simulink library "SlewAndControlConstrained_Controller_lib"  (R2018b)
settings: Solver=VariableStepAuto  StartTime=0.0  StopTime=10.0  RelTol=1e-3
undefined symbols (not defined in the file or in its folder): fswParams
libraries: two_norm x2, aerolibutil x2, dspmtrx3 x1
settings Model: Creator=colem  LastModifiedBy=colem

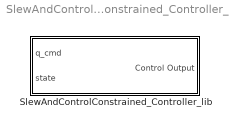
== system SlewAndControlConstrained_Controller_lib ==
  SlewAndControlConstrained_Controller_lib : Subsystem

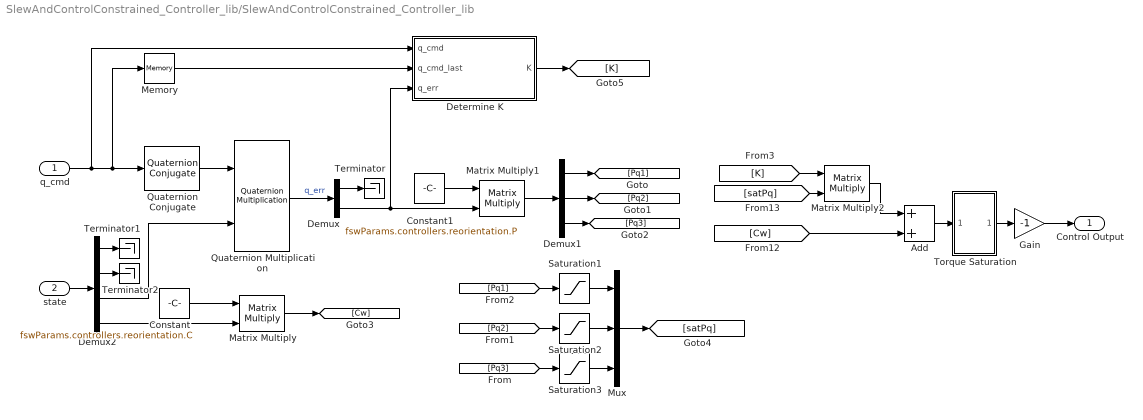
== system SlewAndControlConstrained_Controller_lib/SlewAndControlConstrained_Controller_lib ==
  q_cmd : Inport
  state : Inport  Port=2
  Add : Sum
  Constant : Constant  Value=fswParams.controllers.reorientation.C
  Constant1 : Constant  Value=fswParams.controllers.reorientation.P
  Demux : Demux  Outputs=[1 3]
  Demux1 : Demux  Outputs=3
  Demux2 : Demux  Outputs=[3 3 4 3]
  Determine K : Subsystem
  Gain : Gain  Gain=-1
  Matrix Multiply : Product  Multiplication=Matrix(*)
  Matrix Multiply1 : Product  Multiplication=Matrix(*)
  Matrix Multiply2 : Product  Multiplication=Matrix(*)
  Memory : Memory  InitialCondition=[.5;.5;.5;.5]  InheritSampleTime=on
  Mux : Mux  Inputs=3
  Quaternion Conjugate : aerolibutil/Quaternion Conjugate
      settings: SourceProductName=Aerospace Blockset  SourceProductBaseCode=AE
  Quaternion Multiplication : aerolibutil/Quaternion Multiplication
  Saturation1 : Saturate  UpperLimit=fswParams.controllers.reorientation.saturation  LowerLimit=-fswParams.controllers.reorientation.saturation
  Saturation2 : Saturate  UpperLimit=fswParams.controllers.reorientation.saturation  LowerLimit=-fswParams.controllers.reorientation.saturation
  Saturation3 : Saturate  UpperLimit=fswParams.controllers.reorientation.saturation  LowerLimit=-fswParams.controllers.reorientation.saturation
  Terminator : Terminator
  Terminator1 : Terminator
  Terminator2 : Terminator
  Torque Saturation : Subsystem
  Control Output : Outport
  wires:
  Quaternion Conjugate/1 -> Quaternion Multiplication/1
  Constant1/1 -> Matrix Multiply1/1
  Demux1/3 -> [Pq3]
  Matrix Multiply1/1 -> Demux1/1
  Matrix Multiply/1 -> [Cw]
  Demux1/1 -> [Pq1]
  q_cmd/1 -> Determine K/1(q_cmd), Memory/1, Quaternion Conjugate/1
  Constant/1 -> Matrix Multiply/1
  Demux1/2 -> [Pq2]
  Demux/1 -> Terminator/1
  Quaternion Multiplication/1 -> Demux/1  "q_err"
  Demux/2 -> Matrix Multiply1/2, Determine K/3(q_err)
  [Pq1] -> Saturation1/1
  [Pq2] -> Saturation2/1
  [Pq3] -> Saturation3/1
  [satPq] -> Matrix Multiply2/2
  [Cw] -> Add/2
  Torque Saturation/1(Out1) -> Gain/1
  Gain/1 -> Control Output/1
  Add/1 -> Torque Saturation/1(In1)
  Matrix Multiply2/1 -> Add/1
  state/1 -> Demux2/1
  Demux2/1 -> Terminator1/1
  Demux2/2 -> Terminator2/1
  Demux2/3 -> Quaternion Multiplication/2
  Demux2/4 -> Matrix Multiply/2
  Saturation1/1 -> Mux/1
  Saturation2/1 -> Mux/2
  Saturation3/1 -> Mux/3
  Mux/1 -> [satPq]
  Determine K/1(K) -> [K]
  Memory/1 -> Determine K/2(q_cmd_last)
  [K] -> Matrix Multiply2/1

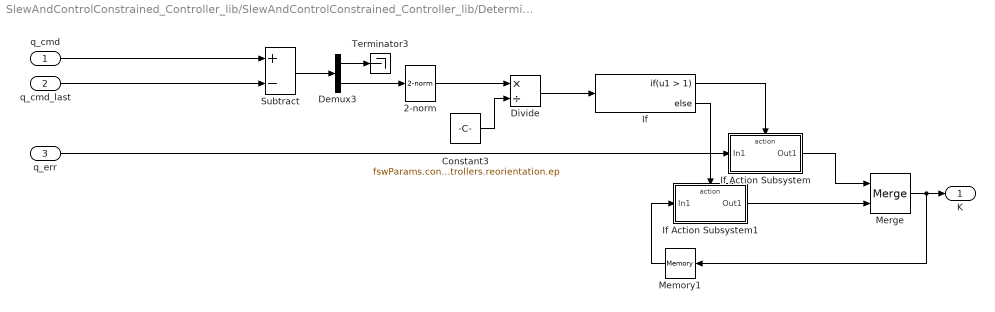
== system SlewAndControlConstrained_Controller_lib/SlewAndControlConstrained_Controller_lib/Determine K ==
  q_cmd : Inport
  q_cmd_last : Inport  Port=2
  q_err : Inport  Port=3
  2-norm : two_norm/2-norm  SystemSampleTime=-1
  Constant3 : Constant  Value=fswParams.controllers.reorientation.ep
  Demux3 : Demux  Outputs=[1 3]
  Divide : Product  Inputs=*/
  If : If  IfExpression=u1 > 1
  If Action Subsystem : Subsystem  TreatAsAtomicUnit=on
  If Action Subsystem1 : Subsystem  TreatAsAtomicUnit=on
  Memory1 : Memory  InitialCondition=fswParams.controllers.reorientation.K_init  InheritSampleTime=on
  Merge : Merge
  Subtract : Sum  Inputs=+-
  Terminator3 : Terminator
  K : Outport
  wires:
  Demux3/2 -> 2-norm/1
  If Action Subsystem/1(Out1) -> Merge/1
  If/1 -> If Action Subsystem/Action
  Divide/1 -> If/1
  q_err/1 -> If Action Subsystem/1(In1)
  2-norm/1 -> Divide/1
  Memory1/1 -> If Action Subsystem1/1(In1)
  Constant3/1 -> Divide/2
  If/2 -> If Action Subsystem1/Action
  If Action Subsystem1/1(Out1) -> Merge/2
  Demux3/1 -> Terminator3/1
  Subtract/1 -> Demux3/1
  Merge/1 -> Memory1/1, K/1
  q_cmd/1 -> Subtract/1
  q_cmd_last/1 -> Subtract/2

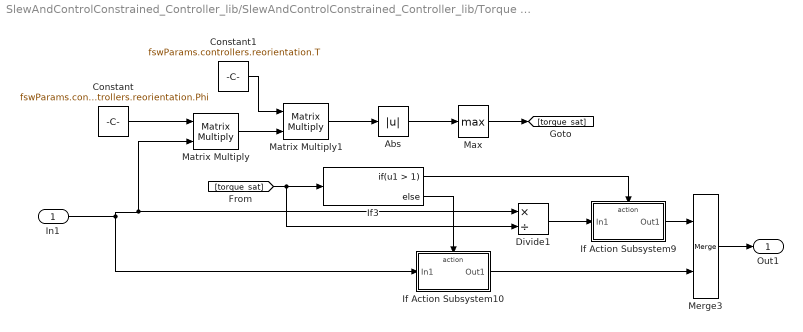
== system SlewAndControlConstrained_Controller_lib/SlewAndControlConstrained_Controller_lib/Torque Saturation ==
  In1 : Inport
  Abs : Abs
  Constant : Constant  Value=fswParams.controllers.reorientation.Phi
  Constant1 : Constant  Value=fswParams.controllers.reorientation.T
  Divide1 : Product  Inputs=*/
  If Action Subsystem10 : Subsystem  TreatAsAtomicUnit=on
  If Action Subsystem9 : Subsystem  TreatAsAtomicUnit=on
  If3 : If  IfExpression=u1 > 1
  Matrix Multiply : Product  Multiplication=Matrix(*)
  Matrix Multiply1 : Product  Multiplication=Matrix(*)
  Max : MinMax  Function=max
  Merge3 : Merge
  Out1 : Outport
  wires:
  If Action Subsystem9/1(Out1) -> Merge3/1
  If3/1 -> If Action Subsystem9/Action
  If3/2 -> If Action Subsystem10/Action
  If Action Subsystem10/1(Out1) -> Merge3/2
  Merge3/1 -> Out1/1
  Divide1/1 -> If Action Subsystem9/1(In1)
  Constant/1 -> Matrix Multiply/1
  In1/1 -> Matrix Multiply/2, Divide1/1, If Action Subsystem10/1(In1)
  Matrix Multiply/1 -> Matrix Multiply1/2
  Constant1/1 -> Matrix Multiply1/1
  Matrix Multiply1/1 -> Abs/1
  Abs/1 -> Max/1
  [torque_sat] -> Divide1/2, If3/1
  Max/1 -> [torque_sat]

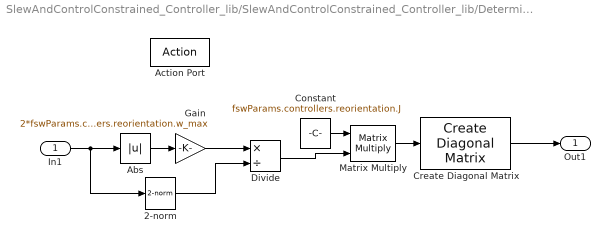
== system SlewAndControlConstrained_Controller_lib/SlewAndControlConstrained_Controller_lib/Determine K/If Action Subsystem ==
  In1 : Inport
  Action Port : ActionPort  ActionType=then
  2-norm : two_norm/2-norm  SystemSampleTime=-1
  Abs : Abs
  Constant : Constant  Value=fswParams.controllers.reorientation.J
  Create Diagonal Matrix : dspmtrx3/Create Diagonal Matrix
      settings: SourceProductName=DSP System Toolbox  SourceProductBaseCode=DS
  Divide : Product  Inputs=*/
  Gain : Gain  Gain=2*fswParams.controllers.reorientation.zeta*fswParams.controllers.reorientation.wn*fswParams.controllers.reorientation.w_max
  Matrix Multiply : Product  Multiplication=Matrix(*)
  Out1 : Outport
  wires:
  In1/1 -> 2-norm/1, Abs/1
  Abs/1 -> Gain/1
  Constant/1 -> Matrix Multiply/1
  2-norm/1 -> Divide/2
  Gain/1 -> Divide/1
  Divide/1 -> Matrix Multiply/2
  Matrix Multiply/1 -> Create Diagonal Matrix/1
  Create Diagonal Matrix/1 -> Out1/1

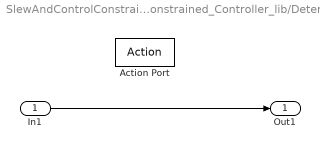
== system SlewAndControlConstrained_Controller_lib/SlewAndControlConstrained_Controller_lib/Determine K/If Action Subsystem1 ==
  In1 : Inport
  Action Port : ActionPort  ActionType=else
  Out1 : Outport
  wires:
  In1/1 -> Out1/1

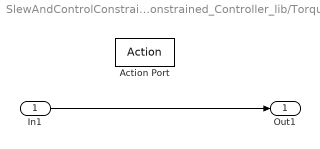
== system SlewAndControlConstrained_Controller_lib/SlewAndControlConstrained_Controller_lib/Torque Saturation/If Action Subsystem10 ==
  In1 : Inport
  Action Port : ActionPort  ActionType=else
  Out1 : Outport
  wires:
  In1/1 -> Out1/1

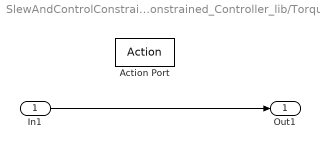
== system SlewAndControlConstrained_Controller_lib/SlewAndControlConstrained_Controller_lib/Torque Saturation/If Action Subsystem9 ==
  In1 : Inport
  Action Port : ActionPort  ActionType=then
  Out1 : Outport
  wires:
  In1/1 -> Out1/1
